simulink model "single_integrator_formation_control"  (R2024a)
settings: Solver=VariableStepAuto  StartTime=0.0  StopTime=5  RelTol=1e-3
settings Model: Creator=LOQ  LastModifiedBy=LOQ

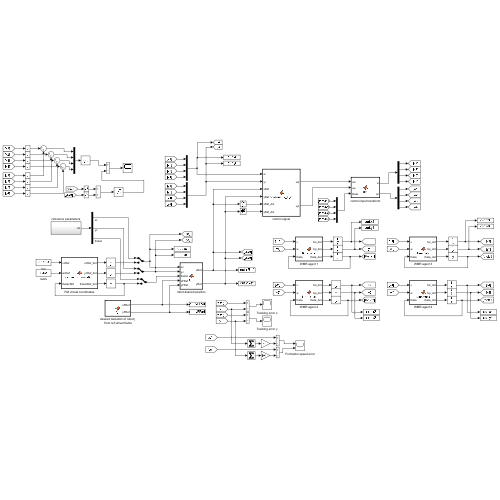
[thumbnail: Simulink's stored preview of the top-level diagram]
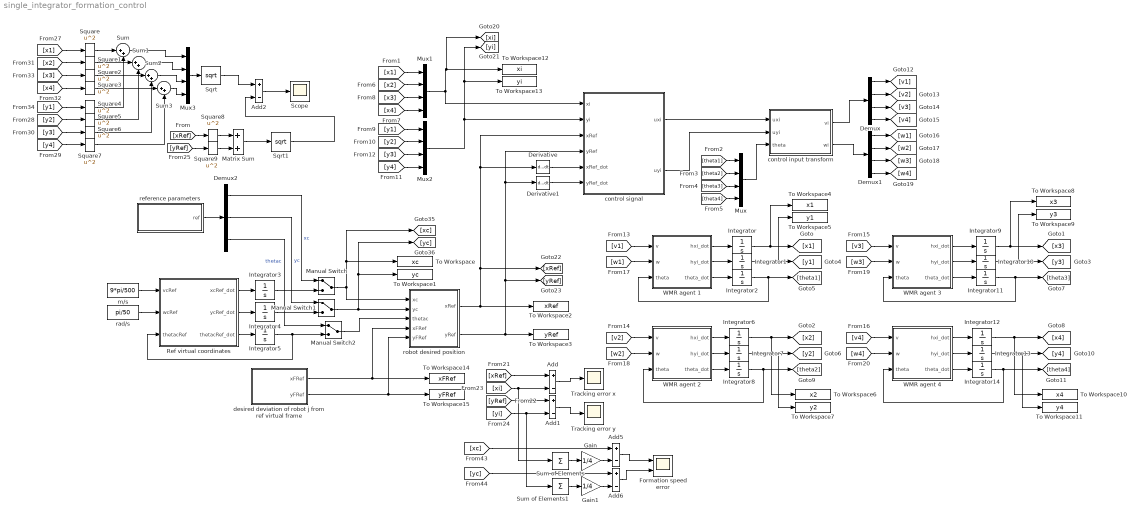
== system single_integrator_formation_control ==
  Add{,1..2,5..6} (5 alike) : Sum  Inputs=+-
  Demux : Demux
  Demux1 : Demux
  Demux2 : Demux  Outputs=3
  Derivative : Derivative
  Derivative1 : Derivative
  Formation speed error : Scope  NumInputPorts=2
  Gain : Gain  Gain=1/4
  Gain1 : Gain  Gain=1/4
  Integrator : Integrator  InitialCondition=0.7
  Integrator1 : Integrator  InitialCondition=0.5
  Integrator10 : Integrator  InitialCondition=0.3
  Integrator11 : Integrator  InitialCondition=-pi/3
  Integrator12 : Integrator  InitialCondition=-0.5
  Integrator13 : Integrator  InitialCondition=0.9
  Integrator14 : Integrator  InitialCondition=pi/4
  Integrator{2..5} (4 alike) : Integrator
  Integrator6 : Integrator  InitialCondition=-0.6
  Integrator7 : Integrator  InitialCondition=0.4
  Integrator8 : Integrator  InitialCondition=pi/2
  Integrator9 : Integrator  InitialCondition=-0.8
  Manual Switch : ManualSwitch
  Manual Switch1 : ManualSwitch
  Manual Switch2 : ManualSwitch
  Matrix Sum : Sum
  Mux{,1..3} (4 alike) : Mux
  Ref virtual coordinates : MATLAB Function  TreatAsAtomicUnit=on
  Scope : Scope
  Sqrt : Sqrt
  Sqrt1 : Sqrt
  Square{,1..9} (10 alike) : Math  Operator=square
  Sum{,1..3} (4 alike) : Sum  Inputs=|++
  Sum of Elements : Sum  Inputs=+
  Sum of Elements1 : Sum  Inputs=+
  To Workspace : ToWorkspace  VariableName=xc  SampleTime=-1
  To Workspace1 : ToWorkspace  VariableName=yc  SampleTime=-1
  To Workspace10 : ToWorkspace  VariableName=x4  SampleTime=-1
  To Workspace11 : ToWorkspace  VariableName=y4  SampleTime=-1
  To Workspace12 : ToWorkspace  VariableName=xi  SampleTime=-1
  To Workspace13 : ToWorkspace  VariableName=yi  SampleTime=-1
  To Workspace14 : ToWorkspace  VariableName=xFRef  SampleTime=-1
  To Workspace15 : ToWorkspace  VariableName=yFRef  SampleTime=-1
  To Workspace2 : ToWorkspace  VariableName=xRef  SampleTime=-1
  To Workspace3 : ToWorkspace  VariableName=yRef  SampleTime=-1
  To Workspace4 : ToWorkspace  VariableName=x1  SampleTime=-1
  To Workspace5 : ToWorkspace  VariableName=y1  SampleTime=-1
  To Workspace6 : ToWorkspace  VariableName=x2  SampleTime=-1
  To Workspace7 : ToWorkspace  VariableName=y2  SampleTime=-1
  To Workspace8 : ToWorkspace  VariableName=x3  SampleTime=-1
  To Workspace9 : ToWorkspace  VariableName=y3  SampleTime=-1
  Tracking error x : Scope
  Tracking error y : Scope
  WMR agent 1 : MATLAB Function  TreatAsAtomicUnit=on
  WMR agent 2 : MATLAB Function  TreatAsAtomicUnit=on
  WMR agent 3 : MATLAB Function  TreatAsAtomicUnit=on
  WMR agent 4 : MATLAB Function  TreatAsAtomicUnit=on
  control input transform : MATLAB Function  TreatAsAtomicUnit=on
  control signal : MATLAB Function  TreatAsAtomicUnit=on
  desired deviation of robot j from ref virtual frame : MATLAB Function  TreatAsAtomicUnit=on
  m/s : Constant  Value=9*pi/500
  rad/s : Constant  Value=pi/50
  reference parameters : Subsystem
  robot desired position : MATLAB Function  TreatAsAtomicUnit=on
  wires:
  m/s/1 -> Ref virtual coordinates/1(vcRef)
  rad/s/1 -> Ref virtual coordinates/2(wcRef)
  WMR agent 1/1(hxi_dot) -> Integrator/1
  WMR agent 1/2(hyi_dot) -> Integrator1/1
  WMR agent 1/3(theta_dot) -> Integrator2/1
  Ref virtual coordinates/1(xcRef_dot) -> Integrator3/1
  Ref virtual coordinates/3(thetacRef_dot) -> Integrator5/1
  Ref virtual coordinates/2(ycRef_dot) -> Integrator4/1
  Integrator5/1 -> Manual Switch2/2, Ref virtual coordinates/3(thetacRef)
  WMR agent 2/2(hyi_dot) -> Integrator7/1
  WMR agent 2/1(hxi_dot) -> Integrator6/1
  WMR agent 2/3(theta_dot) -> Integrator8/1
  WMR agent 3/2(hyi_dot) -> Integrator10/1
  WMR agent 3/1(hxi_dot) -> Integrator9/1
  WMR agent 3/3(theta_dot) -> Integrator11/1
  WMR agent 4/2(hyi_dot) -> Integrator13/1
  WMR agent 4/1(hxi_dot) -> Integrator12/1
  WMR agent 4/3(theta_dot) -> Integrator14/1
  Integrator/1 -> To Workspace4/1, [x1]
  Integrator2/1 -> WMR agent 1/3(theta), [theta1]
  Integrator1/1 -> To Workspace5/1, [y1]
  Integrator8/1 -> WMR agent 2/3(theta), [theta2]
  Integrator11/1 -> WMR agent 3/3(theta), [theta3]
  Integrator14/1 -> WMR agent 4/3(theta), [theta4]
  Mux/1 -> control input transform/3(theta)
  [theta1] -> Mux/1
  [theta2] -> Mux/2
  [theta3] -> Mux/3
  [theta4] -> Mux/4
  Mux1/1 -> [xi], To Workspace12/1, control signal/1(xi)
  [x1] -> Mux1/1
  [x4] -> Mux1/4
  [x2] -> Mux1/2
  [x3] -> Mux1/3
  Mux2/1 -> [yi], To Workspace13/1, control signal/2(yi)
  [y2] -> Mux2/2
  [y1] -> Mux2/1
  [y3] -> Mux2/3
  [y4] -> Mux2/4
  control input transform/1(vi) -> Demux/1
  Demux/1 -> [v1]
  Demux/2 -> [v2]
  Demux/3 -> [v3]
  Demux/4 -> [v4]
  Demux1/3 -> [w3]
  Demux1/2 -> [w2]
  Demux1/4 -> [w4]
  Demux1/1 -> [w1]
  control input transform/2(wi) -> Demux1/1
  control signal/1(uxi) -> control input transform/1(uxi)
  control signal/2(uyi) -> control input transform/2(uyi)
  [v1] -> WMR agent 1/1(v)
  [w1] -> WMR agent 1/2(w)
  [v3] -> WMR agent 3/1(v)
  [w3] -> WMR agent 3/2(w)
  [v4] -> WMR agent 4/1(v)
  [w4] -> WMR agent 4/2(w)
  [v2] -> WMR agent 2/1(v)
  [w2] -> WMR agent 2/2(w)
  desired deviation of robot j from ref virtual frame/1(xFRef) -> To Workspace14/1, robot desired position/4(xFRef)
  desired deviation of robot j from ref virtual frame/2(yFRef) -> To Workspace15/1, robot desired position/5(yFRef)
  Integrator6/1 -> To Workspace6/1, [x2]
  Integrator7/1 -> To Workspace7/1, [y2]
  Integrator9/1 -> To Workspace8/1, [x3]
  Integrator10/1 -> To Workspace9/1, [y3]
  Integrator12/1 -> To Workspace10/1, [x4]
  Integrator13/1 -> To Workspace11/1, [y4]
  [xRef] -> Add/1
  [yRef] -> Add1/1
  [xi] -> Sum of Elements/1, Add/2
  [yi] -> Sum of Elements1/1, Add1/2
  Add/1 -> Tracking error x/1
  Add1/1 -> Tracking error y/1
  robot desired position/1(xRef) -> To Workspace2/1, control signal/3(xRef), Derivative/1, [xRef]
  robot desired position/2(yRef) -> To Workspace3/1, control signal/4(yRef), Derivative1/1, [yRef]
  Derivative/1 -> control signal/5(xRef_dot)
  Derivative1/1 -> control signal/6(yRef_dot)
  Demux2/2 -> Manual Switch1/1  "yc"
  reference parameters/1(ref) -> Demux2/1
  Demux2/3 -> Manual Switch2/1  "thetac"
  Demux2/1 -> Manual Switch/1  "xc"
  Integrator3/1 -> Manual Switch/2
  Integrator4/1 -> Manual Switch1/2
  [x1] -> Square/1
  [x2] -> Square1/1
  [x3] -> Square2/1
  [x4] -> Square3/1
  [y1] -> Square4/1
  [y2] -> Square5/1
  [y3] -> Square6/1
  [y4] -> Square7/1
  Square/1 -> Sum/1
  Square4/1 -> Sum/2
  Square1/1 -> Sum1/1
  Square5/1 -> Sum1/2
  Square2/1 -> Sum2/1
  Square6/1 -> Sum2/2
  Square3/1 -> Sum3/1
  Square7/1 -> Sum3/2
  Sum3/1 -> Mux3/4
  Sum2/1 -> Mux3/3
  Sum1/1 -> Mux3/2
  Sum/1 -> Mux3/1
  Mux3/1 -> Sqrt/1
  [xRef] -> Square8/1
  [yRef] -> Square9/1
  Matrix Sum/1 -> Sqrt1/1
  Add2/1 -> Scope/1
  Sqrt/1 -> Add2/1
  Sqrt1/1 -> Add2/2
  Square8/1 -> Matrix Sum/1
  Square9/1 -> Matrix Sum/2
  Sum of Elements/1 -> Gain/1
  [xc] -> Add5/1
  Gain1/1 -> Add6/2
  Sum of Elements1/1 -> Gain1/1
  Add5/1 -> Formation speed error/1
  [yc] -> Add6/1
  Add6/1 -> Formation speed error/2
  Gain/1 -> Add5/2
  Manual Switch/1 -> [xc], To Workspace/1, robot desired position/1(xc)
  Manual Switch1/1 -> [yc], To Workspace1/1, robot desired position/2(yc)
  Manual Switch2/1 -> robot desired position/3(thetac)

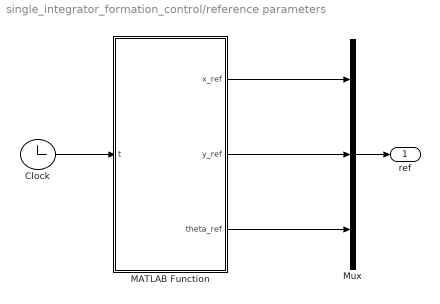
== system single_integrator_formation_control/reference parameters ==
  Clock : Clock
  MATLAB Function : MATLAB Function  TreatAsAtomicUnit=on
  Mux : Mux  Inputs=3
  ref : Outport
  wires:
  Mux/1 -> ref/1
  Clock/1 -> MATLAB Function/1(t)
  MATLAB Function/1(x_ref) -> Mux/1
  MATLAB Function/2(y_ref) -> Mux/2
  MATLAB Function/3(theta_ref) -> Mux/3

== matlab function single_integrator_formation_control/WMR agent 4 ==
  data: v input; hxi_dot output; w input; theta input; hyi_dot output; theta_dot output
function [hxi_dot, hyi_dot, theta_dot] = Kinematic (v,w,theta)

L = 0.1;
R = [cos(theta) -L*sin(theta);
     sin(theta) L*cos(theta);
     0 1];

V = [v; w];

% Output
H = R*V;

hxi_dot = H(1);
hyi_dot = H(2);
theta_dot = H(3);

end

== matlab function single_integrator_formation_control/reference parameters/MATLAB Function ==
  data: x_ref output; y_ref output; theta_ref output; t input
function [x_ref,y_ref,theta_ref] = reference(t)

% curved trajectory
x_ref = -t;
y_ref = sin(0.5*t)+0.5*t+1;
dxRef = -1;
dyRef =  0.5*cos(0.5*t)+0.5;
theta_ref =  atan2(dyRef, dxRef);


end

== matlab function single_integrator_formation_control/WMR agent 1 ==
  data: v input; hxi_dot output; w input; theta input; hyi_dot output; theta_dot output
function [hxi_dot, hyi_dot, theta_dot] = Kinematic (v,w,theta)

L = 0.1;
R = [cos(theta) -L*sin(theta);
     sin(theta) L*cos(theta);
     0 1];

V = [v; w];

% Output
H = R*V;

hxi_dot = H(1);
hyi_dot = H(2);
theta_dot = H(3);

end

== matlab function single_integrator_formation_control/control input transform ==
  data: uxi input; vi output; uyi input; wi output; theta input
function [vi, wi] = fcn(uxi, uyi, theta)

% R = [cos(theta) sin(theta);
%     -sin(theta)/L cos(theta)/L];
% U = [uxi; uyi];
% 
% V = R*U;
% vi = V(1);
% wi = V(2);

L = 0.15; %m
vi = cos(theta) .*uxi + sin(theta) .*uyi;
wi = -sin(theta)/L .*uxi + cos(theta)/L .*uyi; 

end

== matlab function single_integrator_formation_control/desired deviation of robot j from ref virtual frame ==
  data: xFRef output; yFRef output
function [xFRef, yFRef] = fcn ()
% Squared formation

l = 0.6;
j = [1;2;3;4];
% phiRef = pi*[1;1;1;1] - pi/4 * j;
phiRef = pi/2 * (j-1);
xFRef = l*cos(phiRef); 
yFRef = l*sin(phiRef);
          
end

== matlab function single_integrator_formation_control/robot desired position ==
  data: xRef output; yRef output; xc input; yc input; thetac input; xFRef input; yFRef input
function [xRef, yRef] = fcn (xc, yc, thetac, xFRef, yFRef)

% R = [cos(thetac) -sin(thetac);
%      sin(thetac) cos(thetac)];
% rF = [xFRef; yFRef];
% rc = [xc; yc];
% Q = rc + R*rF;
% 
% xRef = Q(1); 
% yRef = Q(2);
          
xRef = xc*[1;1;1;1] + cos(thetac)*xFRef - sin(thetac)*yFRef;
yRef = yc*[1;1;1;1] + sin(thetac)*xFRef + cos(thetac)*yFRef;

% xRef = xc + xFRef;
% yRef = yc + yFRef;
end

== matlab function single_integrator_formation_control/Ref virtual coordinates ==
  data: vcRef input; xcRef_dot output; wcRef input; thetacRef input; ycRef_dot output; thetacRef_dot output
function [xcRef_dot, ycRef_dot, thetacRef_dot] = center_of_formation (vcRef,wcRef,thetacRef)

R = [cos(thetacRef) 0;
     sin(thetacRef) 0;
      0 1];
V = [vcRef; wcRef];

Q = R*V;

xcRef_dot = Q(1); 
ycRef_dot = Q(2);
thetacRef_dot = Q(3);           

end

== matlab function single_integrator_formation_control/control signal ==
  data: uxi output; uyi output; xi input; yi input; xRef input; yRef input; xRef_dot input; yRef_dot input
function [uxi, uyi] = consensus_algo(xi, yi, xRef, yRef, xRef_dot, yRef_dot)

A = [0 1 1 0;
     1 0 0 1;
     0 1 0 0;
     1 0 1 0];
D = diag([2, 2, 1, 2]);
alpha1 = 20;
alpha2 = 20;
alpha3 = 20;
alpha4 = 20;
Q = diag([alpha1, alpha2, alpha3, alpha4]);
L = D - A;

uxi = xRef_dot - (L+Q)*(xi-xRef);
uyi = yRef_dot - (L+Q)*(yi-yRef);
end

== matlab function single_integrator_formation_control/WMR agent 2 ==
  data: v input; hxi_dot output; w input; theta input; hyi_dot output; theta_dot output
function [hxi_dot, hyi_dot, theta_dot] = Kinematic (v,w,theta)

L = 0.1;
R = [cos(theta) -L*sin(theta);
     sin(theta) L*cos(theta);
     0 1];

V = [v; w];

% Output
H = R*V;

hxi_dot = H(1);
hyi_dot = H(2);
theta_dot = H(3);

end

== matlab function single_integrator_formation_control/WMR agent 3 ==
  data: v input; hxi_dot output; w input; theta input; hyi_dot output; theta_dot output
function [hxi_dot, hyi_dot, theta_dot] = Kinematic (v,w,theta)

L = 0.1;
R = [cos(theta) -L*sin(theta);
     sin(theta) L*cos(theta);
     0 1];

V = [v; w];

% Output
H = R*V;

hxi_dot = H(1);
hyi_dot = H(2);
theta_dot = H(3);

end
